simulink model "gm_sampleModel1955_4_sub"  (R2023a)
settings: Solver=VariableStepAuto  StartTime=0.0  StopTime=10.0  RelTol=1e-3
libraries: simulink x5, hdlsllib x1
settings Model: Creator=user1  LastModifiedBy=user1
settings OptimizationCC: BlockReduction=off  ConditionallyExecuteInputs=off
settings DebuggingCC: InheritedTsInSrcMsg=none

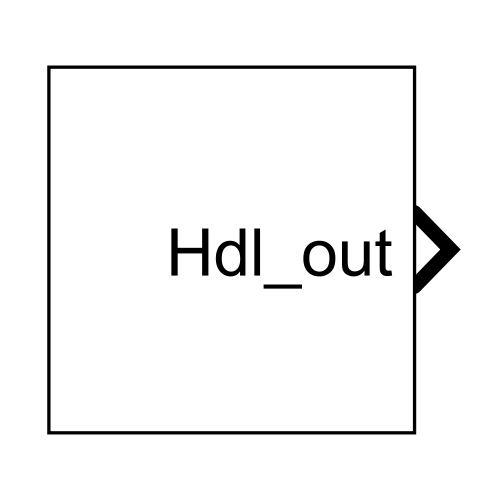
[thumbnail: Simulink's stored preview of the top-level diagram]
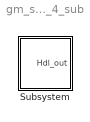
== system gm_sampleModel1955_4_sub ==
  Subsystem : Subsystem

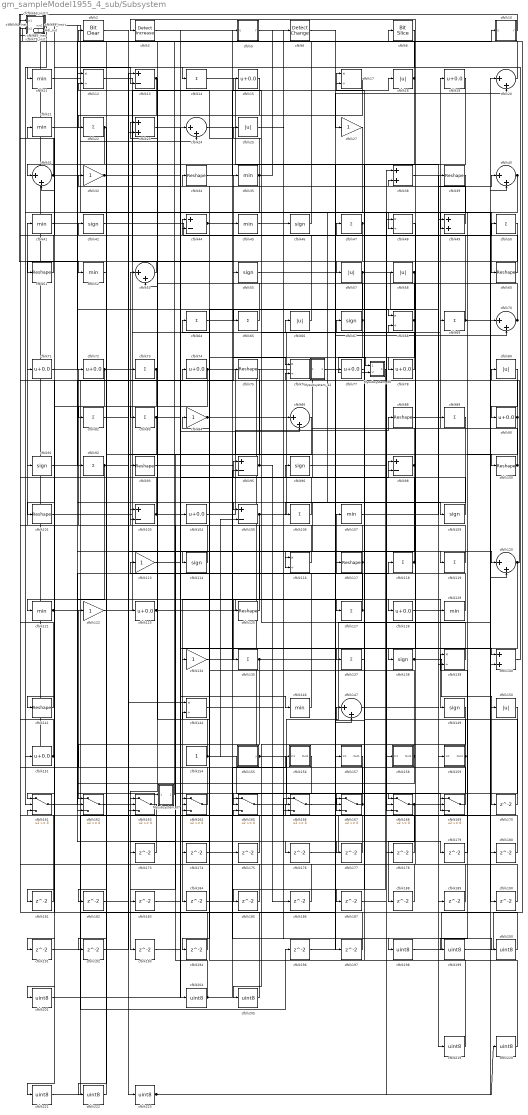
== system gm_sampleModel1955_4_sub/Subsystem ==
  Mysubsystem_30 : Subsystem
  Mysubsystem_37 : Subsystem
  Mysubsystem_42 : Subsystem
  cfblk10 : Subsystem  mask(Detect Rise Positive){vinit=double(0), InputProcessing=Elements as channels (sample based), OutDataTypeStr=uint8}
      mask prompts: vinit "Simulink:masks:InitialCondition_MP"; InputProcessing "Simulink:masks:InputProcessing_MP"; OutDataTypeStr "Simulink:masks:OutputDataType_MP"
      mask help: Simulink:masks:DetectRisePositive_MD
      mask init:
      | InputProcessing = 'Elements as channels (sample based)';
      | OutDataTypeStr = 'uint8';
      | vinit = double(0);
      mask TypeOptions InputProcessing: Simulink:masks:ColumnsAsChannelsFrameBased | Simulink:masks:ElementsAsChannelsSampleBased
      mask TypeOptions OutDataTypeStr: Simulink:masks:uint8 | Simulink:masks:boolean
      mask Display: fprintf('U > 0\n&  NOT\nU/z > 0')
  cfblk{34,39,51,60,75,88,93,100..101,117,125,141} (12 alike) : Reshape
  cfblk{13,44,95,98,103,105} (6 alike) : Sum  Inputs=+-  OutDataTypeStr=uint8
  cfblk{15,19,71..72,74,77..78,90,104,123,128,151} (12 alike) : Bias  Bias=0.0  SaturateOnIntegerOverflow=off
  cfblk{14,22,47,50,64..65,69,73,82..83,89,92,106,118..119,127,135,137} (18 alike) : Sum  Inputs=+  OutDataTypeStr=uint8
  cfblk{11,21,35,41,45,52,107,121,129,146} (10 alike) : MinMax  OutDataTypeStr=uint8
  cfblk{42,46,55,67,91,96,109,114,138,149} (10 alike) : Signum
  cfblk111_inst : Subsystem
  cfblk{27,32,84,113,122,134} (6 alike) : Gain  OutDataTypeStr=uint8
  cfblk115_inst : Subsystem
  cfblk{12,17,48,68,76,116,139,144} (8 alike) : Product  Inputs=*/  OutDataTypeStr=uint8  RndMeth=Zero  SaturateOnIntegerOverflow=on
  cfblk{20,24,31,40,53,70,86,120,147} (9 alike) : Sum  Inputs=|++  OutDataTypeStr=uint8
  cfblk130_inst : Subsystem
  cfblk132_inst : Subsystem
  cfblk{23,38,49,140} (4 alike) : Sum  OutDataTypeStr=uint8
  cfblk145_inst : Subsystem
  cfblk{18,25,57..58,66,80,150} (7 alike) : Abs  OutDataTypeStr=uint8  SaturateOnIntegerOverflow=off
  cfblk152_inst : Subsystem
  cfblk154 : Constant  OutDataTypeStr=uint8  SampleTime=-1
  cfblk155 : Subsystem  mask(Counter Free-Running){NumBits=double(16), tsamp=double(-1)}
      mask prompts: NumBits "Simulink:masks:NumberOfBits_MP"; tsamp "Simulink:masks:SampleTime_MP"
      mask help: Simulink:masks:CounterFreeRunning_MD
  cfblk156 : Subsystem
  cfblk157 : Subsystem
  cfblk158 : Subsystem
  cfblk159 : Subsystem
  cfblk{161..169} (9 alike) : Switch  OutDataTypeStr=uint8  SaturateOnIntegerOverflow=off  InputSameDT=off
  cfblk16_inst : Subsystem
  cfblk{170,173..194,196..197} (25 alike) : Delay  SampleTime=1
  cfblk{198..201,204..205,219..223} (11 alike) : DataTypeConversion  OutDataTypeStr=uint8  SaturateOnIntegerOverflow=off  RndMeth=Floor
  cfblk2 : simulink/Logic and Bit Operations/Bit Clear  iBit=0
      settings: LibrarySourceBlock=|
      | hdlsllib/Logic and Bit
      | Operations/Bit Clear
  cfblk3 : simulink/Logic and Bit Operations/Detect Increase  vinit=0.0  OutDataTypeStr=uint8
      settings: LibrarySourceBlock=|
      | hdlsllib/Logic and Bit
      | Operations/Detect
      | Increase
  cfblk36_inst : Subsystem
  cfblk5 : Subsystem  mask(Detect Fall Negative){vinit=double(0), InputProcessing=Elements as channels (sample based), OutDataTypeStr=uint8}
      mask prompts: vinit "Simulink:masks:InitialCondition_MP"; InputProcessing "Simulink:masks:InputProcessing_MP"; OutDataTypeStr "Simulink:masks:OutputDataType_MP"
      mask help: Simulink:masks:DetectFallNegative_MD
      mask init:
      | InputProcessing = 'Elements as channels (sample based)';
      | OutDataTypeStr = 'uint8';
      | vinit = double(0);
      mask TypeOptions InputProcessing: Simulink:masks:ColumnsAsChannelsFrameBased | Simulink:masks:ElementsAsChannelsSampleBased
      mask TypeOptions OutDataTypeStr: Simulink:masks:uint8 | Simulink:masks:boolean
      mask Display: fprintf('U < 0\n&  NOT\nU/z < 0')
  cfblk59_inst : Subsystem
  cfblk6 : simulink/Logic and Bit Operations/Detect Change  vinit=0  OutDataTypeStr=uint8
      settings: LibrarySourceBlock=|
      | hdlsllib/Logic and Bit
      | Operations/Detect
      | Change
  cfblk62_inst : Subsystem
  cfblk63_inst : Subsystem
  cfblk79_inst : Subsystem
  cfblk8 : hdlsllib/Logic and Bit Operations/Bit Slice  lidx=7  ridx=0
  cfblk85_inst : Subsystem
  cfblk94_inst : Subsystem
  cfblk99_inst : Subsystem
  Hdl_out : Outport  OutDataTypeStr=uint8  SampleTime=1
  wires:
  Mysubsystem_30/1(Out1) -> cfblk185/1
  Mysubsystem_37/1(Out1) -> cfblk111_inst/2(in2)
  Mysubsystem_42/1(Out1) -> Mysubsystem_30/1(In1)
  cfblk10/1(Y) -> cfblk52/1
  cfblk100/1 -> cfblk19/1, cfblk152_inst/1(in1)
  cfblk101/1 -> cfblk17/1
  cfblk103/1 -> cfblk130_inst/2(in2), cfblk104/1, cfblk146/1
  cfblk104/1 -> cfblk88/1
  cfblk105/1 -> cfblk114/1, cfblk184/1, cfblk69/1
  cfblk106/1 -> cfblk42/1
  cfblk107/1 -> cfblk39/1
  cfblk109/1 -> cfblk96/1
  cfblk11/1 -> cfblk60/1
  cfblk111_inst/1(out1) -> cfblk204/1
  cfblk113/1 -> cfblk128/1
  cfblk114/1 -> cfblk63_inst/2(in2)
  cfblk115_inst/1(out1) -> cfblk24/2
  cfblk116/1 -> cfblk72/1
  cfblk117/1 -> cfblk53/1, cfblk132_inst/1(in1), cfblk135/1
  cfblk118/1 -> cfblk95/1, cfblk76/2
  cfblk119/1 -> cfblk84/1
  cfblk12/1 -> cfblk175/1
  cfblk120/1 -> cfblk80/1, cfblk164/3
  cfblk121/1 -> cfblk196/1, Mysubsystem_37/1(In1), cfblk35/1
  cfblk122/1 -> cfblk66/1
  cfblk123/1 -> cfblk23/1, cfblk127/1
  cfblk125/1 -> cfblk41/1
  cfblk127/1 -> cfblk34/1, cfblk107/1
  cfblk128/1 -> cfblk149/1
  cfblk129/1 -> cfblk47/1
  cfblk13/1 -> cfblk23/2, cfblk83/1
  cfblk130_inst/1(out1) -> cfblk13/2
  cfblk132_inst/1(out1) -> cfblk11/1
  cfblk134/1 -> cfblk95/2
  cfblk135/1 -> cfblk77/1, cfblk162/1
  cfblk137/1 -> cfblk17/2
  cfblk138/1 -> cfblk38/2, cfblk170/1
  cfblk139/1 -> cfblk45/1
  cfblk14/1 -> cfblk89/1
  cfblk140/1 -> cfblk14/1
  cfblk141/1 -> cfblk94_inst/2(in2)
  cfblk144/1 -> cfblk179/1
  cfblk145_inst/1(out1) -> cfblk79_inst/2(in2), cfblk168/3, cfblk123/1, cfblk190/1
  cfblk146/1 -> cfblk53/2
  cfblk147/1 -> cfblk219/1
  cfblk149/1 -> cfblk205/1
  cfblk15/1 -> cfblk193/1
  cfblk150/1 -> cfblk174/1
  cfblk151/1 -> cfblk36_inst/2(in2), Hdl_out/1
  cfblk152_inst/1(out1) -> cfblk151/1
  cfblk154/1 -> cfblk169/3, cfblk105/2, cfblk103/1, cfblk113/1, Mysubsystem_42/1(In1)
  cfblk155/1(y) -> cfblk168/1, cfblk167/3
  cfblk156/1(Out1) -> cfblk165/2
  cfblk157/1(Out1) -> cfblk183/1
  cfblk158/1(Out1) -> cfblk162/2, cfblk64/1
  cfblk159/1(Out1) -> cfblk93/1, cfblk168/2
  cfblk16_inst/1(out1) -> cfblk48/2, cfblk197/1
  cfblk161/1 -> cfblk118/1
  cfblk162/1 -> cfblk73/1
  cfblk163/1 -> cfblk161/3
  cfblk164/1 -> cfblk122/1
  cfblk165/1 -> cfblk20/1
  cfblk166/1 -> cfblk167/1
  cfblk167/1 -> cfblk59_inst/2(in2), cfblk92/1
  cfblk168/1 -> cfblk189/1, cfblk188/1
  cfblk169/1 -> cfblk91/1
  cfblk17/1 -> cfblk22/1
  cfblk170/1 -> cfblk48/1
  cfblk173/1 -> cfblk62_inst/1(in1)
  cfblk174/1 -> cfblk167/2
  cfblk175/1 -> cfblk94_inst/1(in1)
  cfblk176/1 -> cfblk120/2
  cfblk177/1 -> cfblk165/1
  cfblk178/1 -> cfblk79_inst/1(in1)
  cfblk179/1 -> cfblk139/1
  cfblk18/1 -> cfblk132_inst/2(in2), cfblk187/1
  cfblk180/1 -> cfblk165/3
  cfblk181/1 -> cfblk59_inst/1(in1)
  cfblk182/1 -> cfblk166/2
  cfblk183/1 -> cfblk98/1
  cfblk184/1 -> cfblk166/1
  cfblk185/1 -> cfblk44/1
  cfblk186/1 -> cfblk16_inst/2(in2)
  cfblk187/1 -> cfblk38/1
  cfblk188/1 -> cfblk145_inst/1(in1)
  cfblk189/1 -> cfblk68/2
  cfblk19/1 -> cfblk161/1
  cfblk190/1 -> cfblk85_inst/2(in2)
  cfblk191/1 -> cfblk70/1
  cfblk192/1 -> cfblk13/1
  cfblk193/1 -> cfblk24/1
  cfblk194/1 -> cfblk115_inst/1(in1)
  cfblk196/1 -> cfblk20/2
  cfblk197/1 -> cfblk99_inst/2(in2)
  cfblk198/1 -> cfblk150/1
  cfblk199/1 -> cfblk3/1
  cfblk2/1 -> cfblk223/1
  cfblk20/1 -> cfblk99_inst/1(in1)
  cfblk200/1 -> cfblk71/1
  cfblk201/1 -> cfblk5/1(U)
  cfblk204/1 -> cfblk103/2, cfblk156/1(In1)
  cfblk205/1 -> cfblk111_inst/1(in1)
  cfblk21/1 -> cfblk176/1
  cfblk219/1 -> cfblk144/2
  cfblk22/1 -> cfblk182/1, cfblk181/1
  cfblk220/1 -> cfblk147/1
  cfblk221/1 -> cfblk147/2
  cfblk222/1 -> cfblk2/1
  cfblk223/1 -> cfblk220/1, cfblk180/1, cfblk178/1
  cfblk23/1 -> cfblk105/1
  cfblk24/1 -> cfblk117/1
  cfblk25/1 -> cfblk166/3
  cfblk27/1 -> cfblk106/1
  cfblk3/1 -> cfblk198/1
  cfblk31/1 -> cfblk63_inst/1(in1), cfblk158/1(In1)
  cfblk32/1 -> cfblk86/2, cfblk137/1
  cfblk34/1 -> cfblk18/1
  cfblk35/1 -> cfblk221/1, cfblk12/2, cfblk6/1
  cfblk36_inst/1(out1) -> cfblk163/1
  cfblk38/1 -> cfblk159/1(In1)
  cfblk39/1 -> cfblk161/2
  cfblk40/1 -> cfblk49/2, cfblk169/1
  cfblk41/1 -> cfblk116/2
  cfblk42/1 -> cfblk50/1
  cfblk44/1 -> cfblk140/1, cfblk76/1
  cfblk45/1 -> cfblk46/1
  cfblk46/1 -> cfblk145_inst/2(in2)
  cfblk47/1 -> cfblk163/2, cfblk121/1
  cfblk48/1 -> cfblk138/1
  cfblk49/1 -> cfblk12/1
  cfblk5/1(Y) -> cfblk200/1
  cfblk50/1 -> cfblk57/1
  cfblk51/1 -> cfblk152_inst/2(in2)
  cfblk52/1 -> cfblk32/1
  cfblk53/1 -> cfblk51/1
  cfblk55/1 -> cfblk70/2
  cfblk57/1 -> cfblk169/2, cfblk164/2, cfblk65/1
  cfblk58/1 -> cfblk78/1, cfblk194/1
  cfblk59_inst/1(out1) -> cfblk109/1
  cfblk6/1 -> cfblk27/1
  cfblk60/1 -> cfblk36_inst/1(in1)
  cfblk62_inst/1(out1) -> cfblk85_inst/1(in1), cfblk31/2
  cfblk63_inst/1(out1) -> cfblk162/3
  cfblk64/1 -> cfblk140/2
  cfblk65/1 -> cfblk55/1
  cfblk66/1 -> cfblk21/1
  cfblk67/1 -> cfblk164/1, cfblk115_inst/2(in2)
  cfblk68/1 -> cfblk16_inst/1(in1), cfblk134/1
  cfblk69/1 -> cfblk8/1, cfblk40/2
  cfblk70/1 -> cfblk25/1, cfblk130_inst/1(in1)
  cfblk71/1 -> cfblk10/1(U)
  cfblk72/1 -> cfblk141/1, cfblk119/1
  cfblk73/1 -> cfblk101/1, cfblk82/1
  cfblk74/1 -> cfblk201/1, cfblk157/1(In1)
  cfblk75/1 -> cfblk173/1
  cfblk76/1 -> Mysubsystem_30/2(U)
  cfblk77/1 -> cfblk58/1
  cfblk78/1 -> cfblk15/1
  cfblk79_inst/1(out1) -> cfblk125/1
  cfblk8/1 -> cfblk31/1
  cfblk80/1 -> cfblk90/1
  cfblk82/1 -> cfblk144/1
  cfblk83/1 -> cfblk67/1, cfblk192/1
  cfblk84/1 -> cfblk86/1, cfblk177/1
  cfblk85_inst/1(out1) -> cfblk129/1
  cfblk86/1 -> cfblk222/1
  cfblk88/1 -> cfblk40/1
  cfblk89/1 -> cfblk116/1
  cfblk90/1 -> cfblk75/1, cfblk49/1, cfblk199/1
  cfblk91/1 -> cfblk74/1
  cfblk92/1 -> cfblk100/1, cfblk191/1
  cfblk93/1 -> cfblk98/2
  cfblk94_inst/1(out1) -> cfblk120/1
  cfblk95/1 -> cfblk44/2, cfblk186/1
  cfblk96/1 -> cfblk139/2
  cfblk98/1 -> cfblk62_inst/2(in2), cfblk163/3
  cfblk99_inst/1(out1) -> cfblk68/1

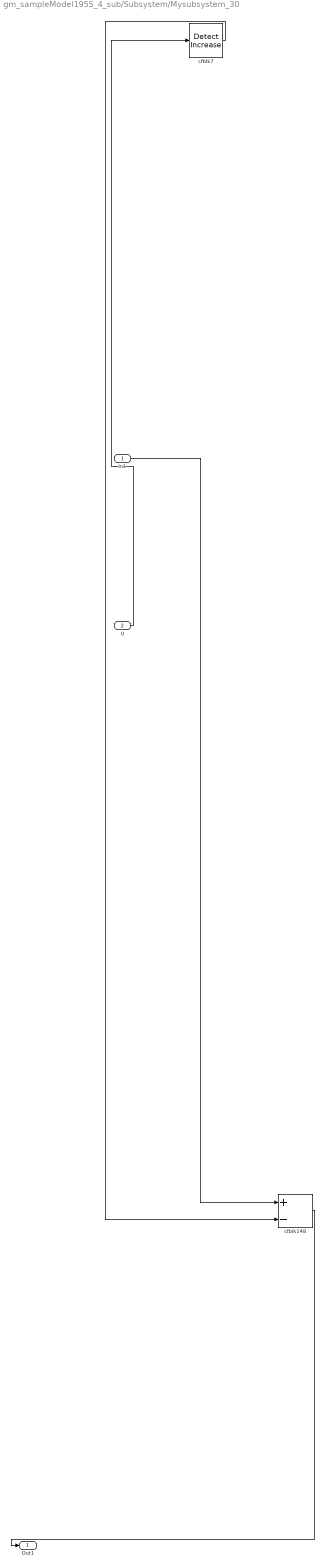
== system gm_sampleModel1955_4_sub/Subsystem/Mysubsystem_30 ==
  In1 : Inport  OutDataTypeStr=uint8  PortDimensions=1  SampleTime=1
  U : Inport  Port=2  OutDataTypeStr=uint8  PortDimensions=1  SampleTime=1
  cfblk148 : Sum  Inputs=+-
  cfblk7 : simulink/Logic and Bit Operations/Detect Increase  vinit=0.0  OutDataTypeStr=boolean
      settings: LibrarySourceBlock=|
      | hdlsllib/Logic and Bit
      | Operations/Detect
      | Increase
  Out1 : Outport  SampleTime=1
  wires:
  In1/1 -> cfblk148/1
  U/1 -> cfblk7/1
  cfblk148/1 -> Out1/1
  cfblk7/1 -> cfblk148/2

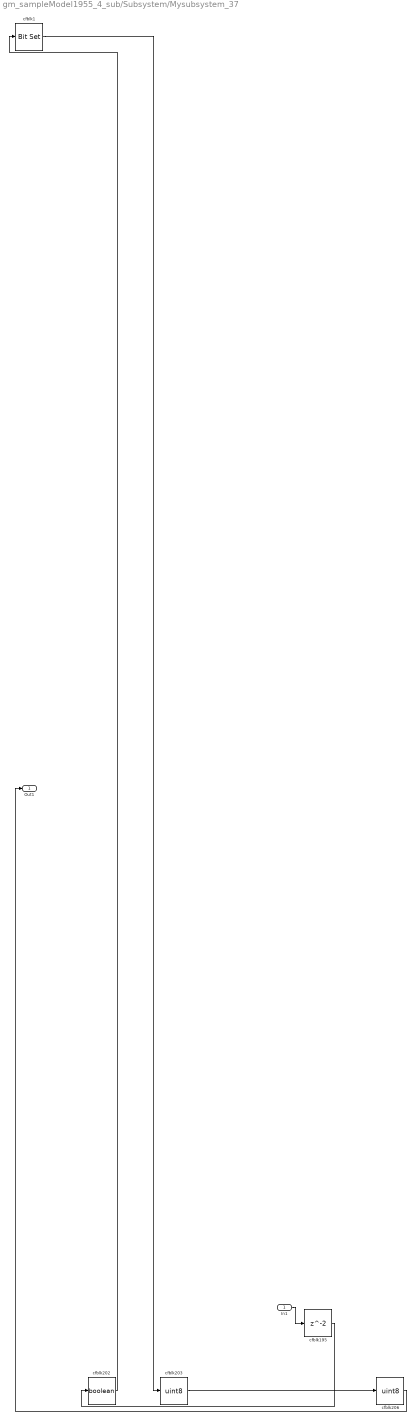
== system gm_sampleModel1955_4_sub/Subsystem/Mysubsystem_37 ==
  In1 : Inport  OutDataTypeStr=uint8  PortDimensions=1  SampleTime=1
  cfblk1 : simulink/Logic and Bit Operations/Bit Set  iBit=0
      settings: LibrarySourceBlock=|
      | hdlsllib/Logic and Bit
      | Operations/Bit Set
  cfblk195 : Delay  SampleTime=1
  cfblk202 : DataTypeConversion  OutDataTypeStr=boolean  SaturateOnIntegerOverflow=off  RndMeth=Floor
  cfblk203 : DataTypeConversion  OutDataTypeStr=uint8  SaturateOnIntegerOverflow=off  RndMeth=Floor
  cfblk206 : DataTypeConversion  OutDataTypeStr=uint8  SaturateOnIntegerOverflow=off  RndMeth=Floor
  Out1 : Outport  SampleTime=1
  wires:
  In1/1 -> cfblk195/1
  cfblk1/1 -> cfblk203/1
  cfblk195/1 -> cfblk202/1
  cfblk202/1 -> cfblk1/1
  cfblk203/1 -> cfblk206/1
  cfblk206/1 -> Out1/1

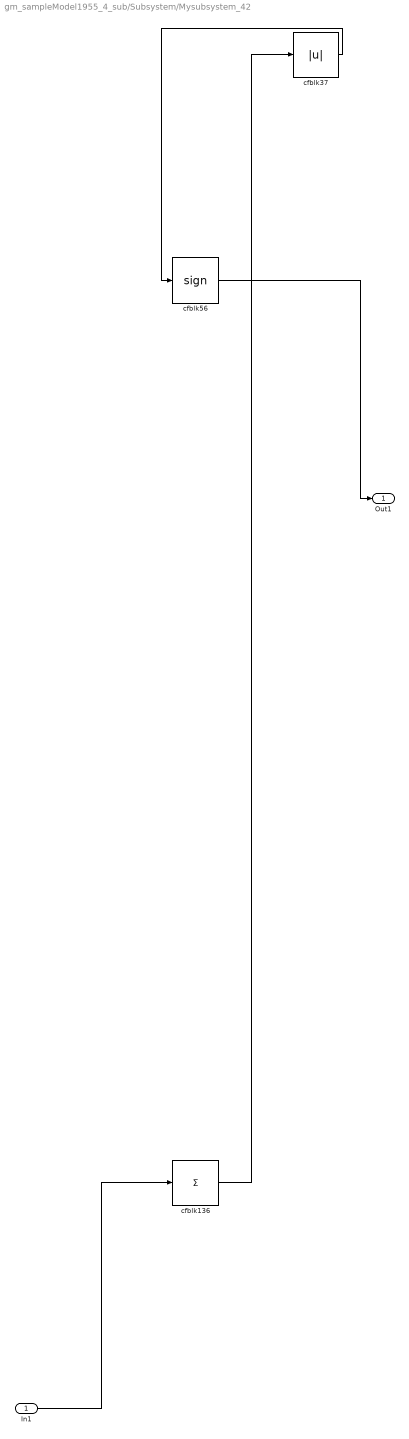
== system gm_sampleModel1955_4_sub/Subsystem/Mysubsystem_42 ==
  In1 : Inport  OutDataTypeStr=uint8  PortDimensions=1  SampleTime=1
  cfblk136 : Sum  Inputs=+
  cfblk37 : Abs  SaturateOnIntegerOverflow=off
  cfblk56 : Signum
  Out1 : Outport  SampleTime=1
  wires:
  In1/1 -> cfblk136/1
  cfblk136/1 -> cfblk37/1
  cfblk37/1 -> cfblk56/1
  cfblk56/1 -> Out1/1

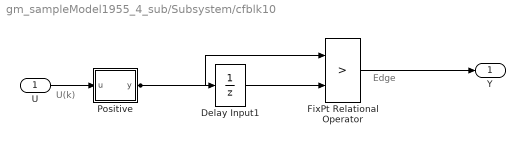
== system gm_sampleModel1955_4_sub/Subsystem/cfblk10 ==
  note: U(k)
  note: Edge
  U : Inport  OutDataTypeStr=uint8  SampleTime=1
  Delay Input1 : UnitDelay  Description=Store in Global RAM  DisableCoverage=on  InitialCondition=vinit  SampleTime=-1  HasFrameUpgradeWarning=on
  FixPt Relational Operator : RelationalOperator  Operator=>  OutDataTypeStr=fixdt(0, 8)  ZeroCross=off  InputSameDT=off
  Positive : Subsystem  mask(Compare To Zero){relop=>, OutDataTypeStr=boolean, ZeroCross=off}
      mask prompts: relop "Simulink:masks:Operator_MP"; OutDataTypeStr "Simulink:masks:OutputDataType_MP"; ZeroCross "Simulink:masks:EnableZerocrossingDetection_MP"
      mask help: Simulink:masks:CompareToZero_MD
      mask init:
      | OutDataTypeStr = 'boolean';
      | ZeroCross = 'off';
      | blkName = 'sampleModel1955_4_sub/Subsystem/cfblk10/Positive';
      | relop = '>';
      | setValue = 'boolean';
      mask TypeOptions relop: == | ~= | < | <= | >= | >
      mask TypeOptions OutDataTypeStr: Simulink:masks:uint8 | Simulink:masks:boolean
      mask Callback ZeroCross: sl('zeroCrossEnable', gcbh);
      mask Display: disp([relop,' 0'])
  Y : Outport  SampleTime=1
  wires:
  U/1 -> Positive/1(u)
  Delay Input1/1 -> FixPt Relational Operator/2
  FixPt Relational Operator/1 -> Y/1
  Positive/1(y) -> FixPt Relational Operator/1, Delay Input1/1

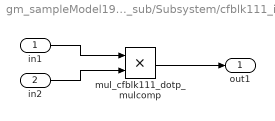
== system gm_sampleModel1955_4_sub/Subsystem/cfblk111_inst ==
  in1 : Inport  OutDataTypeStr=uint8  SampleTime=1
  in2 : Inport  Port=2  OutDataTypeStr=uint8  SampleTime=1
  mul_cfblk111_dotp_mulcomp : Product  Inputs=**  OutDataTypeStr=uint8  SampleTime=1
  out1 : Outport  OutDataTypeStr=uint8  SampleTime=1
  wires:
  in1/1 -> mul_cfblk111_dotp_mulcomp/1
  in2/1 -> mul_cfblk111_dotp_mulcomp/2
  mul_cfblk111_dotp_mulcomp/1 -> out1/1

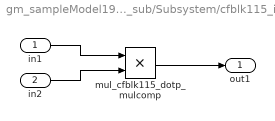
== system gm_sampleModel1955_4_sub/Subsystem/cfblk115_inst ==
  in1 : Inport  OutDataTypeStr=uint8  SampleTime=1
  in2 : Inport  Port=2  OutDataTypeStr=uint8  SampleTime=1
  mul_cfblk115_dotp_mulcomp : Product  Inputs=**  OutDataTypeStr=uint8  SampleTime=1
  out1 : Outport  OutDataTypeStr=uint8  SampleTime=1
  wires:
  in1/1 -> mul_cfblk115_dotp_mulcomp/1
  in2/1 -> mul_cfblk115_dotp_mulcomp/2
  mul_cfblk115_dotp_mulcomp/1 -> out1/1

== system gm_sampleModel1955_4_sub/Subsystem/cfblk130_inst ==
  in1 : Inport  OutDataTypeStr=uint8  SampleTime=1
  in2 : Inport  Port=2  OutDataTypeStr=uint8  SampleTime=1
  mul_cfblk130_dotp_mulcomp : Product  Inputs=**  OutDataTypeStr=uint8  SampleTime=1
  out1 : Outport  OutDataTypeStr=uint8  SampleTime=1
  wires:
  in1/1 -> mul_cfblk130_dotp_mulcomp/1
  in2/1 -> mul_cfblk130_dotp_mulcomp/2
  mul_cfblk130_dotp_mulcomp/1 -> out1/1

== system gm_sampleModel1955_4_sub/Subsystem/cfblk132_inst ==
  in1 : Inport  OutDataTypeStr=uint8  SampleTime=1
  in2 : Inport  Port=2  OutDataTypeStr=uint8  SampleTime=1
  mul_cfblk132_dotp_mulcomp : Product  Inputs=**  OutDataTypeStr=uint8  SampleTime=1
  out1 : Outport  OutDataTypeStr=uint8  SampleTime=1
  wires:
  in1/1 -> mul_cfblk132_dotp_mulcomp/1
  in2/1 -> mul_cfblk132_dotp_mulcomp/2
  mul_cfblk132_dotp_mulcomp/1 -> out1/1

== system gm_sampleModel1955_4_sub/Subsystem/cfblk145_inst ==
  in1 : Inport  OutDataTypeStr=uint8  SampleTime=1
  in2 : Inport  Port=2  OutDataTypeStr=uint8  SampleTime=1
  mul_cfblk145_dotp_mulcomp : Product  Inputs=**  OutDataTypeStr=uint8  SampleTime=1
  out1 : Outport  OutDataTypeStr=uint8  SampleTime=1
  wires:
  in1/1 -> mul_cfblk145_dotp_mulcomp/1
  in2/1 -> mul_cfblk145_dotp_mulcomp/2
  mul_cfblk145_dotp_mulcomp/1 -> out1/1

== system gm_sampleModel1955_4_sub/Subsystem/cfblk152_inst ==
  in1 : Inport  OutDataTypeStr=uint8  SampleTime=1
  in2 : Inport  Port=2  OutDataTypeStr=uint8  SampleTime=1
  mul_cfblk152_dotp_mulcomp : Product  Inputs=**  OutDataTypeStr=uint8  SampleTime=1
  out1 : Outport  OutDataTypeStr=uint8  SampleTime=1
  wires:
  in1/1 -> mul_cfblk152_dotp_mulcomp/1
  in2/1 -> mul_cfblk152_dotp_mulcomp/2
  mul_cfblk152_dotp_mulcomp/1 -> out1/1

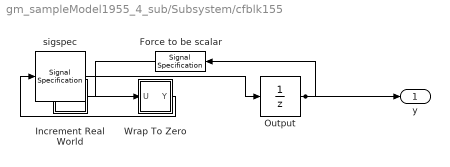
== system gm_sampleModel1955_4_sub/Subsystem/cfblk155 ==
  Force to be scalar : SignalSpecification  DisableCoverage=on  Dimensions=1
  Increment Real World : Subsystem  mask(Real World Value Increment){}
      mask help: Simulink:masks:RealWorldValueIncrement_MD
      mask Display: disp('V++')
  Output : UnitDelay  InitialCondition=0.0  SampleTime=tsamp  HasFrameUpgradeWarning=on
  Wrap To Zero : Subsystem  mask(Wrap To Zero){Threshold=double(65535)}
      mask prompts: Threshold "Simulink:masks:Threshold_MP"
      mask help: Simulink:masks:WrapToZero_MD
  sigspec : SignalSpecification  OutDataTypeStr=uint16  Dimensions=1
  y : Outport  SampleTime=1
  wires:
  Force to be scalar/1 -> Increment Real World/1(u)
  Increment Real World/1(y) -> Wrap To Zero/1(U)
  Output/1 -> Force to be scalar/1, y/1
  Wrap To Zero/1(Y) -> sigspec/1
  sigspec/1 -> Output/1

== system gm_sampleModel1955_4_sub/Subsystem/cfblk156 ==
  In1 : Inport  OutDataTypeStr=uint8  PortDimensions=1  SampleTime=1
  Out1 : Outport  SampleTime=1
  wires:
  In1/1 -> Out1/1

== system gm_sampleModel1955_4_sub/Subsystem/cfblk157 ==
  In1 : Inport  OutDataTypeStr=uint8  PortDimensions=1  SampleTime=1
  Out1 : Outport  SampleTime=1
  wires:
  In1/1 -> Out1/1

== system gm_sampleModel1955_4_sub/Subsystem/cfblk158 ==
  In1 : Inport  OutDataTypeStr=uint8  PortDimensions=1  SampleTime=1
  Out1 : Outport  SampleTime=1
  wires:
  In1/1 -> Out1/1

== system gm_sampleModel1955_4_sub/Subsystem/cfblk159 ==
  In1 : Inport  OutDataTypeStr=uint8  PortDimensions=1  SampleTime=1
  Out1 : Outport  SampleTime=1
  wires:
  In1/1 -> Out1/1

== system gm_sampleModel1955_4_sub/Subsystem/cfblk16_inst ==
  in1 : Inport  OutDataTypeStr=uint8  SampleTime=1
  in2 : Inport  Port=2  OutDataTypeStr=uint8  SampleTime=1
  mul_cfblk16_dotp_mulcomp : Product  Inputs=**  OutDataTypeStr=uint8  SampleTime=1
  out1 : Outport  OutDataTypeStr=uint8  SampleTime=1
  wires:
  in1/1 -> mul_cfblk16_dotp_mulcomp/1
  in2/1 -> mul_cfblk16_dotp_mulcomp/2
  mul_cfblk16_dotp_mulcomp/1 -> out1/1

== system gm_sampleModel1955_4_sub/Subsystem/cfblk36_inst ==
  in1 : Inport  OutDataTypeStr=uint8  SampleTime=1
  in2 : Inport  Port=2  OutDataTypeStr=uint8  SampleTime=1
  mul_cfblk36_dotp_mulcomp : Product  Inputs=**  OutDataTypeStr=uint8  SampleTime=1
  out1 : Outport  OutDataTypeStr=uint8  SampleTime=1
  wires:
  in1/1 -> mul_cfblk36_dotp_mulcomp/1
  in2/1 -> mul_cfblk36_dotp_mulcomp/2
  mul_cfblk36_dotp_mulcomp/1 -> out1/1

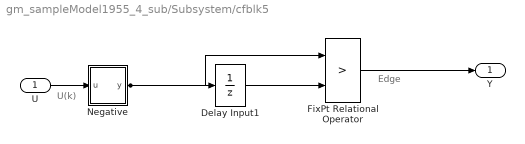
== system gm_sampleModel1955_4_sub/Subsystem/cfblk5 ==
  note: U(k)
  note: Edge
  U : Inport  OutDataTypeStr=uint8  SampleTime=1
  Delay Input1 : UnitDelay  Description=Store in Global RAM  DisableCoverage=on  InitialCondition=vinit  SampleTime=-1  HasFrameUpgradeWarning=on
  FixPt Relational Operator : RelationalOperator  Operator=>  OutDataTypeStr=fixdt(0, 8)  ZeroCross=off  InputSameDT=off
  Negative : Subsystem  mask(Compare To Zero){relop=<, OutDataTypeStr=boolean, ZeroCross=off}
      mask prompts: relop "Simulink:masks:Operator_MP"; OutDataTypeStr "Simulink:masks:OutputDataType_MP"; ZeroCross "Simulink:masks:EnableZerocrossingDetection_MP"
      mask help: Simulink:masks:CompareToZero_MD
      mask init:
      | OutDataTypeStr = 'boolean';
      | ZeroCross = 'off';
      | blkName = 'sampleModel1955_4_sub/Subsystem/cfblk5/Negative';
      | relop = '<';
      | setValue = 'boolean';
      mask TypeOptions relop: == | ~= | < | <= | >= | >
      mask TypeOptions OutDataTypeStr: Simulink:masks:uint8 | Simulink:masks:boolean
      mask Callback ZeroCross: sl('zeroCrossEnable', gcbh);
      mask Display: disp([relop,' 0'])
  Y : Outport  SampleTime=1
  wires:
  U/1 -> Negative/1(u)
  Delay Input1/1 -> FixPt Relational Operator/2
  FixPt Relational Operator/1 -> Y/1
  Negative/1(y) -> FixPt Relational Operator/1, Delay Input1/1

== system gm_sampleModel1955_4_sub/Subsystem/cfblk59_inst ==
  in1 : Inport  OutDataTypeStr=uint8  SampleTime=1
  in2 : Inport  Port=2  OutDataTypeStr=uint8  SampleTime=1
  mul_cfblk59_dotp_mulcomp : Product  Inputs=**  OutDataTypeStr=uint8  SampleTime=1
  out1 : Outport  OutDataTypeStr=uint8  SampleTime=1
  wires:
  in1/1 -> mul_cfblk59_dotp_mulcomp/1
  in2/1 -> mul_cfblk59_dotp_mulcomp/2
  mul_cfblk59_dotp_mulcomp/1 -> out1/1

== system gm_sampleModel1955_4_sub/Subsystem/cfblk62_inst ==
  in1 : Inport  OutDataTypeStr=uint8  SampleTime=1
  in2 : Inport  Port=2  OutDataTypeStr=uint8  SampleTime=1
  mul_cfblk62_dotp_mulcomp : Product  Inputs=**  OutDataTypeStr=uint8  SampleTime=1
  out1 : Outport  OutDataTypeStr=uint8  SampleTime=1
  wires:
  in1/1 -> mul_cfblk62_dotp_mulcomp/1
  in2/1 -> mul_cfblk62_dotp_mulcomp/2
  mul_cfblk62_dotp_mulcomp/1 -> out1/1

== system gm_sampleModel1955_4_sub/Subsystem/cfblk63_inst ==
  in1 : Inport  OutDataTypeStr=uint8  SampleTime=1
  in2 : Inport  Port=2  OutDataTypeStr=uint8  SampleTime=1
  mul_cfblk63_dotp_mulcomp : Product  Inputs=**  OutDataTypeStr=uint8  SampleTime=1
  out1 : Outport  OutDataTypeStr=uint8  SampleTime=1
  wires:
  in1/1 -> mul_cfblk63_dotp_mulcomp/1
  in2/1 -> mul_cfblk63_dotp_mulcomp/2
  mul_cfblk63_dotp_mulcomp/1 -> out1/1

== system gm_sampleModel1955_4_sub/Subsystem/cfblk79_inst ==
  in1 : Inport  OutDataTypeStr=uint8  SampleTime=1
  in2 : Inport  Port=2  OutDataTypeStr=uint8  SampleTime=1
  mul_cfblk79_dotp_mulcomp : Product  Inputs=**  OutDataTypeStr=uint8  SampleTime=1
  out1 : Outport  OutDataTypeStr=uint8  SampleTime=1
  wires:
  in1/1 -> mul_cfblk79_dotp_mulcomp/1
  in2/1 -> mul_cfblk79_dotp_mulcomp/2
  mul_cfblk79_dotp_mulcomp/1 -> out1/1

== system gm_sampleModel1955_4_sub/Subsystem/cfblk85_inst ==
  in1 : Inport  OutDataTypeStr=uint8  SampleTime=1
  in2 : Inport  Port=2  OutDataTypeStr=uint8  SampleTime=1
  mul_cfblk85_dotp_mulcomp : Product  Inputs=**  OutDataTypeStr=uint8  SampleTime=1
  out1 : Outport  OutDataTypeStr=uint8  SampleTime=1
  wires:
  in1/1 -> mul_cfblk85_dotp_mulcomp/1
  in2/1 -> mul_cfblk85_dotp_mulcomp/2
  mul_cfblk85_dotp_mulcomp/1 -> out1/1

== system gm_sampleModel1955_4_sub/Subsystem/cfblk94_inst ==
  in1 : Inport  OutDataTypeStr=uint8  SampleTime=1
  in2 : Inport  Port=2  OutDataTypeStr=uint8  SampleTime=1
  mul_cfblk94_dotp_mulcomp : Product  Inputs=**  OutDataTypeStr=uint8  SampleTime=1
  out1 : Outport  OutDataTypeStr=uint8  SampleTime=1
  wires:
  in1/1 -> mul_cfblk94_dotp_mulcomp/1
  in2/1 -> mul_cfblk94_dotp_mulcomp/2
  mul_cfblk94_dotp_mulcomp/1 -> out1/1

== system gm_sampleModel1955_4_sub/Subsystem/cfblk99_inst ==
  in1 : Inport  OutDataTypeStr=uint8  SampleTime=1
  in2 : Inport  Port=2  OutDataTypeStr=uint8  SampleTime=1
  mul_cfblk99_dotp_mulcomp : Product  Inputs=**  OutDataTypeStr=uint8  SampleTime=1
  out1 : Outport  OutDataTypeStr=uint8  SampleTime=1
  wires:
  in1/1 -> mul_cfblk99_dotp_mulcomp/1
  in2/1 -> mul_cfblk99_dotp_mulcomp/2
  mul_cfblk99_dotp_mulcomp/1 -> out1/1

== system gm_sampleModel1955_4_sub/Subsystem/cfblk10/Positive ==
  u : Inport  OutDataTypeStr=uint8  SampleTime=1
  Compare : RelationalOperator  Operator=>  OutDataTypeStr=boolean  ZeroCross=off
  Constant : Constant  DisableCoverage=on  Value=0  OutDataTypeStr=Inherit: Inherit via back propagation  SampleTime=-1  PreserveConstantTs=on
  y : Outport  SampleTime=1
  wires:
  u/1 -> Compare/1
  Compare/1 -> y/1
  Constant/1 -> Compare/2

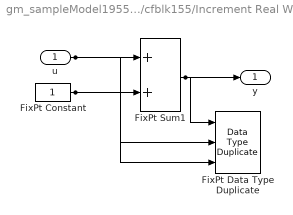
== system gm_sampleModel1955_4_sub/Subsystem/cfblk155/Increment Real World ==
  u : Inport  OutDataTypeStr=uint16  SampleTime=1
  FixPt Constant : Constant  DisableCoverage=on  OutDataTypeStr=Inherit: Inherit via back propagation  SampleTime=-1
  FixPt Data Type Duplicate : DataTypeDuplicate  DisableCoverage=on  NumInputPorts=3
  FixPt Sum1 : Sum  InputSameDT=on  OutDataTypeStr=Inherit: Inherit via back propagation  LockScale=on
  y : Outport  SampleTime=1
  wires:
  u/1 -> FixPt Sum1/1, FixPt Data Type Duplicate/2
  FixPt Constant/1 -> FixPt Sum1/2, FixPt Data Type Duplicate/3
  FixPt Sum1/1 -> FixPt Data Type Duplicate/1, y/1

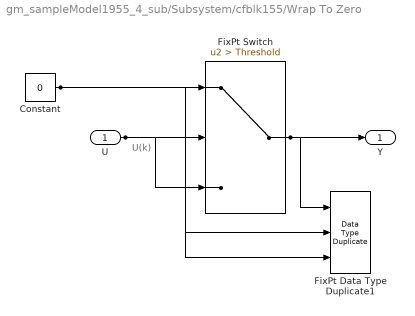
== system gm_sampleModel1955_4_sub/Subsystem/cfblk155/Wrap To Zero ==
  note: U(k)
  U : Inport  OutDataTypeStr=uint16  SampleTime=1
  Constant : Constant  DisableCoverage=on  Value=0  OutDataTypeStr=Inherit: Inherit via back propagation  SampleTime=-1
  FixPt Data Type Duplicate1 : DataTypeDuplicate  DisableCoverage=on  NumInputPorts=3
  FixPt Switch : Switch  Criteria=u2 > Threshold  Threshold=Threshold  OutDataTypeStr=Inherit: Inherit via back propagation  ZeroCross=off  SaturateOnIntegerOverflow=off  InputSameDT=off
  Y : Outport  SampleTime=1
  wires:
  U/1 -> FixPt Switch/3, FixPt Switch/2, FixPt Data Type Duplicate1/2
  Constant/1 -> FixPt Switch/1, FixPt Data Type Duplicate1/3
  FixPt Switch/1 -> FixPt Data Type Duplicate1/1, Y/1

== system gm_sampleModel1955_4_sub/Subsystem/cfblk5/Negative ==
  u : Inport  OutDataTypeStr=uint8  SampleTime=1
  Compare : RelationalOperator  Operator=<  OutDataTypeStr=boolean  ZeroCross=off
  Constant : Constant  DisableCoverage=on  Value=0  OutDataTypeStr=Inherit: Inherit via back propagation  SampleTime=-1  PreserveConstantTs=on
  y : Outport  SampleTime=1
  wires:
  u/1 -> Compare/1
  Compare/1 -> y/1
  Constant/1 -> Compare/2
